simulink model "chap5_2sim"  (Simulink 8.8)
settings: Solver=ode45  StartTime=0.0  StopTime=100.0  RelTol=1e-3
settings Model: SuppressorTable=22 serialization::archive 11 0 3 0 0 0 0 0  Creator=guoshaopan  LastModifiedBy=guoshaopan
settings DataIOCC: LimitDataPoints=off  SaveFormat=Dataset  SignalLoggingSaveFormat=Dataset
settings OptimizationCC: LifeSpan=auto
settings DebuggingCC: UnderspecifiedInitializationDetection=Simplified  MergeDetectMultiDrivingBlocksExec=error  FcnCallInpInsideContextMsg=error  StateNameClashWarn=none  SFUnexpectedBacktrackingDiag=error  SFNoUnconditionalDefaultTransitionDiag=error  SFExecutionAtInitializationDiag=warning
settings HardwareCC: ProdBitPerPointer=64  ProdBitPerSizeT=64  ProdBitPerPtrDiffT=64  ProdLargestAtomicFloat=Float  ProdIntDivRoundTo=Zero  ProdEndianess=LittleEndian  ProdWordSize=64  ProdHWDeviceType=Intel->x86-64 (Windows64)
settings ModelReferenceCC: PropagateSignalLabelsOutOfModel=on
settings GRTTargetCC: TargetLangStandard=C99 (ISO)  GeneratePreprocessorConditionals=Use local settings  CombineOutputUpdateFcns=on  GRTInterface=off
settings ConfigComp: CovMetricSettings=dwe  CovHtmlReporting=off  CovSaveCumulativeToWorkspaceVar=off  CovSaveSingleToWorkspaceVar=off  CovExternalEMLEnable=on

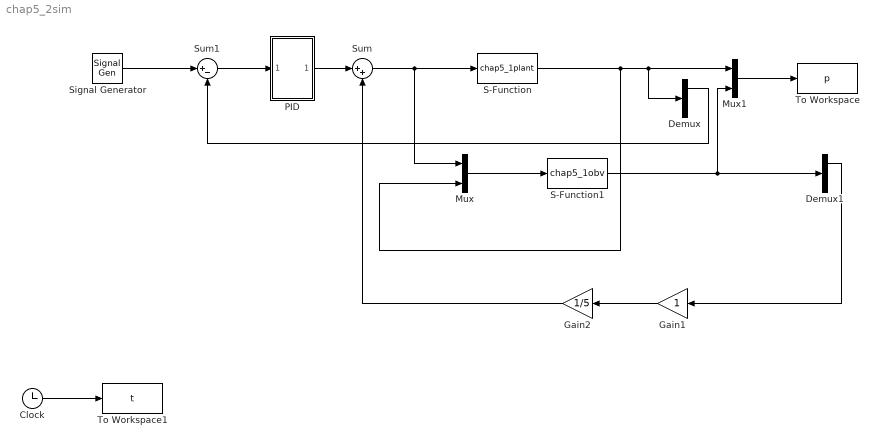
== system chap5_2sim ==
  Clock : Clock
  Demux : Demux  Outputs=2
  Demux1 : Demux  Outputs=2
  Gain1 : Gain
  Gain2 : Gain  Gain=1/5
  Mux : Mux  Inputs=2
  Mux1 : Mux  Inputs=2
  PID : Subsystem
  S-Function : S-Function  FunctionName=chap5_1plant  SFunctionDeploymentMode=off  EnableBusSupport=off
  S-Function1 : S-Function  FunctionName=chap5_1obv  SFunctionDeploymentMode=off  EnableBusSupport=off
  Signal Generator : SignalGenerator  Units=rad/sec
  Sum : Sum  Inputs=|++
  Sum1 : Sum  Inputs=|+-
  To Workspace : ToWorkspace  VariableName=p  SampleTime=-1
  To Workspace1 : ToWorkspace  VariableName=t  SampleTime=-1
  wires:
  Mux/1 -> S-Function1/1
  S-Function/1 -> Demux/1, Mux1/1, Mux/2
  S-Function1/1 -> Demux1/1, Mux1/2
  Mux1/1 -> To Workspace/1
  Clock/1 -> To Workspace1/1
  Sum/1 -> Mux/1, S-Function/1
  PID/1(Out1) -> Sum/1
  Sum1/1 -> PID/1(In1)
  Demux/1 -> Sum1/2
  Signal Generator/1 -> Sum1/1
  Demux1/1 -> Gain1/1
  Gain1/1 -> Gain2/1
  Gain2/1 -> Sum/2

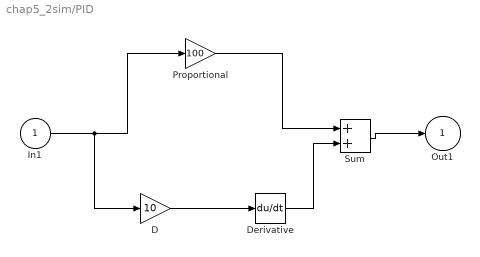
== system chap5_2sim/PID ==
  In1 : Inport
  D : Gain  Gain=10
  Derivative : Derivative
  Proportional : Gain  Gain=100
  Sum : Sum
  Out1 : Outport
  wires:
  Proportional/1 -> Sum/1
  In1/1 -> D/1, Proportional/1
  D/1 -> Derivative/1
  Sum/1 -> Out1/1
  Derivative/1 -> Sum/2
